simulink model "SinglePhase_NLCurrent_compensation"  (R2017b)
settings: Solver=ode4  StartTime=0.0  StopTime=simend  FixedStep=ts  RelTol=1e-3
values from neighbouring files (symbols this model uses):
  B = BT(:,1:size(B1,2))    [SinglePhase_NLCurrent_compensation_parameter.m]
  gamma = zeros(Hp*n,Hp*d)    [mpc_matrixSetup.m]
  hp = num    (= 1000)    [SinglePhase_NLCurrent_compensation_parameter.m]
  hu = hp    (= 1000)    [SinglePhase_NLCurrent_compensation_parameter.m]
  mtd = 3    [SinglePhase_NLCurrent_compensation_parameter.m]
  num = 1000    [SinglePhase_NLCurrent_compensation_parameter.m]
  psi = zeros(Hp*n,n)    [mpc_matrixSetup.m]
  Q = QPv    [SinglePhase_NLCurrent_compensation_parameter.m]
  R = 1*10^(+5-0)*eye(hu*size(B,2))    [SinglePhase_NLCurrent_compensation_parameter.m]
  ref = ref(:)    [SinglePhase_NLCurrent_compensation_parameter.m]
  Rline = 1    [SinglePhase_NLCurrent_compensation_parameter.m]
  SQ = Pv    [SinglePhase_NLCurrent_compensation_parameter.m]
  SR = chol(R)    [SinglePhase_NLCurrent_compensation_parameter.m]
  theta = zeros(Hp*n,Hu*m)    [mpc_matrixSetup.m]
  ts = 1/f/num    (= 2e-05)    [SinglePhase_NLCurrent_compensation_parameter.m]
  ups = zeros(Hp*n,m)    [mpc_matrixSetup.m]
undefined symbols (not defined in the file or in its folder): A
libraries: fl_lib x37, nesl_utility x21, simulink x4, powerlib_meascontrol x1
settings Model: PauseTimes=0.02  Creator=Weihe  LastModifiedBy=Weihe

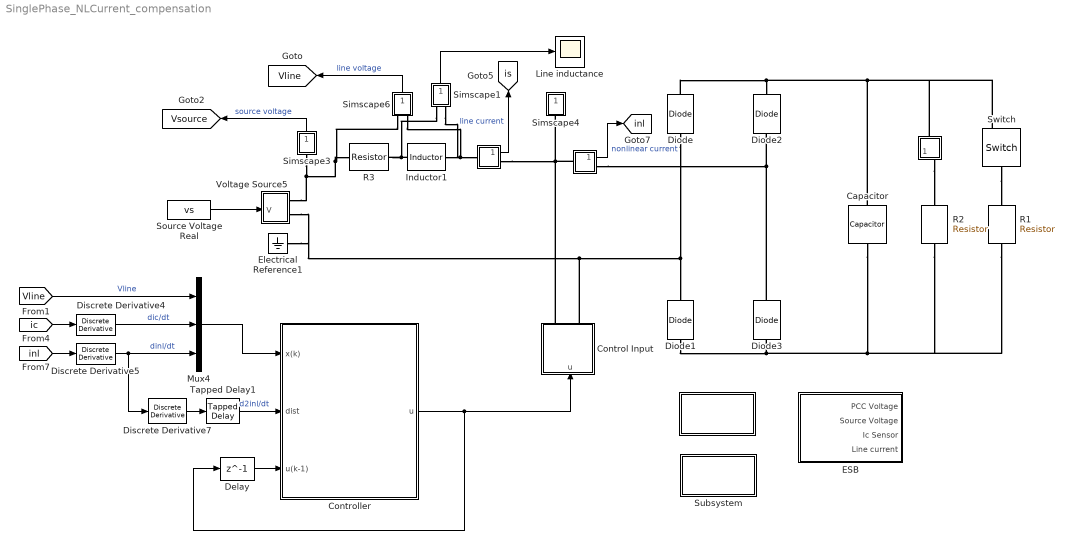
== system SinglePhase_NLCurrent_compensation ==
  " " : Subsystem
      mask Display: disp('A')
  "     " : Subsystem
      mask Display: disp('A')
  "      " : Subsystem
      mask Display: disp('A')
  "           " : Subsystem
      mask Display: disp('THD Calculation')
  Capacitor : fl_lib/Electrical/Electrical Elements/Capacitor  c=5e-3 F  r=1e-6 Ohm  g=0 1/Ohm  i_specify=off  i_priority=None  i=0 A  i_nominal_specify=off  i_nominal_unit=A  i_nominal_value=1  v_specify=off  v_priority=None  v=0 V  v_nominal_specify=off  v_nominal_unit=V  v_nominal_value=1  vc_specify=off  vc_priority=High  vc=0 V  vc_nominal_specify=off  vc_nominal_unit=V  vc_nominal_value=1
  Control Input : Subsystem
  Controller : Subsystem
  Delay : Delay  DelayLength=1
  Diode{,1..3} (4 alike) : fl_lib/Electrical/Electrical Elements/Diode  Vf=0.6 V  Ron=0.3 Ohm  Goff=1e-8 1/Ohm  i_specify=off  i_priority=None  i=0 A  i_nominal_specify=off  i_nominal_unit=A  i_nominal_value=1  v_specify=off  v_priority=None  v=0 V  v_nominal_specify=off  v_nominal_unit=V  v_nominal_value=1
  Discrete Derivative4 : simulink/Discrete/Discrete Derivative  gainval=1e-0  ICPrevScaledInput=0.0  OutMin=[]  OutMax=[]  OutDataType=fixdt(1, 16)  OutScaling=2^-10  DoSatur=off
  Discrete Derivative5 : simulink/Discrete/Discrete Derivative  gainval=1e-0  ICPrevScaledInput=0.0  OutMin=[]  OutMax=[]  OutDataType=fixdt(1, 16)  OutScaling=2^-10  DoSatur=off
  Discrete Derivative7 : simulink/Discrete/Discrete Derivative  gainval=1.0  ICPrevScaledInput=0.0  OutMin=[]  OutMax=[]  OutDataType=fixdt(1, 16)  OutScaling=2^-10  DoSatur=off
  ESB : Subsystem
  Electrical Reference1 : fl_lib/Electrical/Electrical Elements/Electrical Reference
  Inductor1 : fl_lib/Electrical/Electrical Elements/Inductor  l=Lline H  r=0 Ohm  g=1e-9 1/Ohm  i_specify=off  i_priority=None  i=0 A  i_nominal_specify=off  i_nominal_unit=A  i_nominal_value=1  v_specify=off  v_priority=None  v=0 V  v_nominal_specify=off  v_nominal_unit=V  v_nominal_value=1  i_L_specify=off  i_L_priority=High  i_L=0 A  i_L_nominal_specify=off  i_L_nominal_unit=A  i_L_nominal_value=1
  Line inductance : Scope
  Mux4 : Mux  Inputs=3
  R1 : fl_lib/Electrical/Electrical Elements/Resistor  R=10 Ohm  i_specify=off  i_priority=High  i=0 A  i_nominal_specify=off  i_nominal_unit=A  i_nominal_value=1  v_specify=off  v_priority=High  v=0 V  v_nominal_specify=off  v_nominal_unit=V  v_nominal_value=1
  R2 : fl_lib/Electrical/Electrical Elements/Resistor  R=10 Ohm  i_specify=off  i_priority=High  i=0 A  i_nominal_specify=off  i_nominal_unit=A  i_nominal_value=1  v_specify=off  v_priority=High  v=0 V  v_nominal_specify=off  v_nominal_unit=V  v_nominal_value=1
  R3 : fl_lib/Electrical/Electrical Elements/Resistor  R=Rline Ohm  i_specify=off  i_priority=High  i=0 A  i_nominal_specify=off  i_nominal_unit=A  i_nominal_value=1  v_specify=off  v_priority=High  v=0 V  v_nominal_specify=off  v_nominal_unit=V  v_nominal_value=1
  Simscape1 : Subsystem
      mask Display: disp('V')
  Simscape3 : Subsystem
      mask Display: disp('V')
  Simscape4 : Subsystem
      mask Display: disp('V')
  Simscape6 : Subsystem
      mask Display: disp('V')
  Source Voltage Real : FromWorkspace  VariableName=vs  SampleTime=ts  Interpolate=off  OutputAfterFinalValue=Holding final value
  Subsystem : Subsystem
      mask Display: disp('Scopes')
  Switch : fl_lib/Electrical/Electrical Elements/Switch  R_closed=0.01 Ohm  G_open=1e-8 1/Ohm  Threshold=0  i_specify=off  i_priority=None  i=0 A  i_nominal_specify=off  i_nominal_unit=A  i_nominal_value=1  v_specify=off  v_priority=None  v=0 V  v_nominal_specify=off  v_nominal_unit=V  v_nominal_value=1
      settings: SourceProductName=Simscape
  Tapped Delay1 : simulink/Discrete/Tapped Delay  vinit=0.0  samptime=ts  NumDelays=num  DelayOrder=Oldest  includeCurrent=off
  Voltage Source5 : Subsystem
  tag scope: Vline=global, Vsource=global, inl=global, is=global
  wires:
  Source Voltage Real/1 -> Voltage Source5/1(V)
  " "/1(Out1) -> [is]  "line current"
  Discrete Derivative4/1 -> Mux4/2  "dic/dt"
  Discrete Derivative5/1 -> Discrete Derivative7/1, Mux4/3  "dinl/dt"
  "      "/1(Out1) -> [inl]  "nonlinear current"
  Controller/1(u) -> Control Input/1(u), Delay/1
  Mux4/1 -> Controller/1(x(k))
  Tapped Delay1/1 -> Controller/2(dist)  "d2inl/dt"
  Delay/1 -> Controller/3(u(k-1))
  Discrete Derivative7/1 -> Tapped Delay1/1
  Simscape6/1(Out) -> [Vline]  "line voltage"
  [Vline] -> Mux4/1  "Vline"
  [ic] -> Discrete Derivative4/1
  [inl] -> Discrete Derivative5/1
  Simscape3/1(Out) -> [Vsource]  "source voltage"
  Simscape1/1(Out) -> Line inductance/1
  connections:
  Voltage Source5/RConn1 -- Simscape6/LConn1 -- R3/LConn1 -- Simscape3/LConn1
  Diode/LConn1 -- Diode1/RConn1 -- Control Input/RConn2 -- Electrical Reference1/LConn1 -- Voltage Source5/RConn2
  Diode3/RConn1 -- "      "/RConn1 -- Diode2/LConn1
  Diode/RConn1 -- Switch/RConn2 -- "     "/LConn1 -- Capacitor/LConn1 -- Diode2/RConn1
  Diode1/LConn1 -- R1/RConn1 -- R2/RConn1 -- Capacitor/RConn1 -- Diode3/LConn1
  "     "/RConn1 -- R2/LConn1
  Inductor1/RConn1 -- Simscape1/LConn2 -- Simscape6/LConn2 -- " "/LConn1
  Inductor1/LConn1 -- Simscape1/LConn1 -- R3/RConn1
  "      "/LConn1 -- Control Input/RConn1 -- " "/RConn1 -- Simscape4/LConn1
  Switch/LConn1 -- R1/LConn1

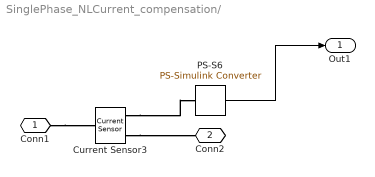
== system SinglePhase_NLCurrent_compensation/  ==
  Current Sensor3 : fl_lib/Electrical/Electrical Sensors/Current Sensor  mask(Current Sensor){}
  PS-S6 : nesl_utility/PS-Simulink Converter  PhysicalDomain=network_engine_domain  SubClassName=ps_output  LeftPortType=input  RightPortType=output  PseudoPeriodic=off  Frequencies=[]  Unit=A  AffineConversion=off
  Conn1 : PMIOPort  Port=1  Side=Left
  Conn2 : PMIOPort  Port=2  Side=Right
  Out1 : Outport
  wires:
  PS-S6/1 -> Out1/1
  connections:
  Current Sensor3/RConn2 -- Conn2/RConn1
  Conn1/RConn1 -- Current Sensor3/LConn1
  Current Sensor3/RConn1 -- PS-S6/LConn1

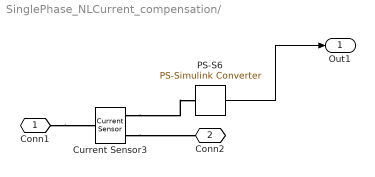
== system SinglePhase_NLCurrent_compensation/      ==
  Current Sensor3 : fl_lib/Electrical/Electrical Sensors/Current Sensor  mask(Current Sensor){}
  PS-S6 : nesl_utility/PS-Simulink Converter  PhysicalDomain=network_engine_domain  SubClassName=ps_output  LeftPortType=input  RightPortType=output  PseudoPeriodic=off  Frequencies=[]  Unit=A  AffineConversion=off
  Conn1 : PMIOPort  Port=1  Side=Left
  Conn2 : PMIOPort  Port=2  Side=Right
  Out1 : Outport
  wires:
  PS-S6/1 -> Out1/1
  connections:
  Current Sensor3/RConn2 -- Conn2/RConn1
  Conn1/RConn1 -- Current Sensor3/LConn1
  Current Sensor3/RConn1 -- PS-S6/LConn1

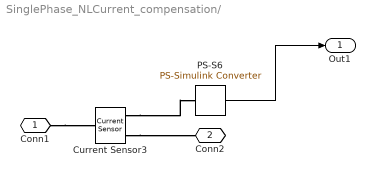
== system SinglePhase_NLCurrent_compensation/       ==
  Current Sensor3 : fl_lib/Electrical/Electrical Sensors/Current Sensor  mask(Current Sensor){}
  PS-S6 : nesl_utility/PS-Simulink Converter  PhysicalDomain=network_engine_domain  SubClassName=ps_output  LeftPortType=input  RightPortType=output  PseudoPeriodic=off  Frequencies=[]  Unit=A  AffineConversion=off
  Conn1 : PMIOPort  Port=1  Side=Left
  Conn2 : PMIOPort  Port=2  Side=Right
  Out1 : Outport
  wires:
  PS-S6/1 -> Out1/1
  connections:
  Current Sensor3/RConn2 -- Conn2/RConn1
  Conn1/RConn1 -- Current Sensor3/LConn1
  Current Sensor3/RConn1 -- PS-S6/LConn1

== system SinglePhase_NLCurrent_compensation/            ==
  Display : Display
  THD : powerlib_meascontrol/Measurements/THD  Freq=f  Ts=ts
  THD Vline : Scope
  wires:
  THD/1 -> Display/1, THD Vline/1
  [is] -> THD/1

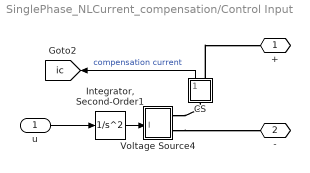
== system SinglePhase_NLCurrent_compensation/Control Input ==
  u : Inport
  CS : Subsystem
      mask Display: disp('A')
  "Integrator, Second-Order1" : SecondOrderIntegrator  ShowOutput=x
  Voltage Source4 : Subsystem
  + : PMIOPort  Port=1  Side=Right
  - : PMIOPort  Port=2  Side=Right
  tag scope: ic=global
  wires:
  "Integrator, Second-Order1"/1 -> Voltage Source4/1(I)
  u/1 -> "Integrator, Second-Order1"/1
  CS/1(Out1) -> [ic]  "compensation current"
  connections:
  Voltage Source4/RConn1 -- CS/LConn1
  CS/RConn1 -- +/RConn1
  Voltage Source4/RConn2 -- -/RConn1

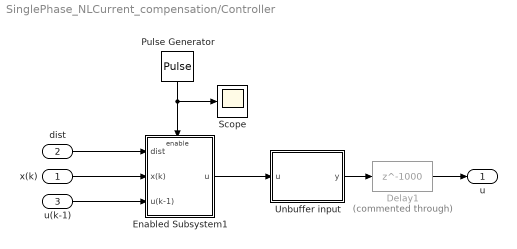
== system SinglePhase_NLCurrent_compensation/Controller ==
  x(k) : Inport
  dist : Inport  Port=2
  u(k-1) : Inport  Port=3
  Delay1 : Delay  Commented=through  DelayLength=1000
  Enabled Subsystem1 : Subsystem  TreatAsAtomicUnit=on
  Pulse Generator : DiscretePulseGenerator  Period=num  SampleTime=ts
  Scope : Scope
  Unbuffer input : MATLAB Function  TreatAsAtomicUnit=on  SystemSampleTime=ts
  u : Outport
  wires:
  Pulse Generator/1 -> Enabled Subsystem1/Enable, Scope/1
  dist/1 -> Enabled Subsystem1/1(dist)
  Delay1/1 -> u/1
  x(k)/1 -> Enabled Subsystem1/2(x(k))
  u(k-1)/1 -> Enabled Subsystem1/3(u(k-1))
  Enabled Subsystem1/1(u) -> Unbuffer input/1(u)
  Unbuffer input/1(y) -> Delay1/1

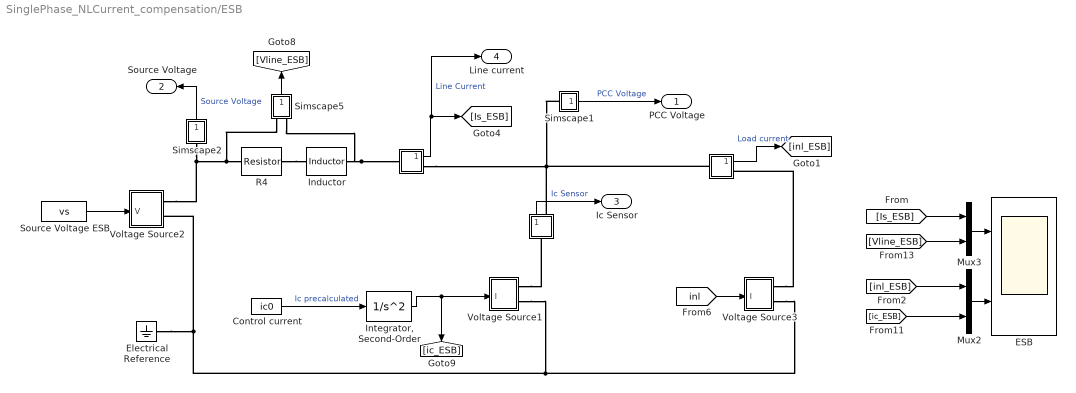
== system SinglePhase_NLCurrent_compensation/ESB ==
  "  " : Subsystem
      mask Display: disp('A')
  "   " : Subsystem
      mask Display: disp('A')
  "    " : Subsystem
      mask Display: disp('A')
  Control current : FromWorkspace  VariableName=ic0  SampleTime=ts  Interpolate=off  OutputAfterFinalValue=Holding final value
  ESB : Scope  NumInputPorts=2
  Electrical Reference : fl_lib/Electrical/Electrical Elements/Electrical Reference
  Inductor : fl_lib/Electrical/Electrical Elements/Inductor  l=Lline H  r=0 Ohm  g=1e-9 1/Ohm  i_specify=off  i_priority=None  i=0 A  i_nominal_specify=off  i_nominal_unit=A  i_nominal_value=1  v_specify=off  v_priority=None  v=0 V  v_nominal_specify=off  v_nominal_unit=V  v_nominal_value=1  i_L_specify=off  i_L_priority=High  i_L=0 A  i_L_nominal_specify=off  i_L_nominal_unit=A  i_L_nominal_value=1
  "Integrator, Second-Order" : SecondOrderIntegrator  ShowOutput=x
  Mux2 : Mux  Inputs=2
  Mux3 : Mux  Inputs=2
  R4 : fl_lib/Electrical/Electrical Elements/Resistor  R=Rline Ohm  i_specify=off  i_priority=High  i=0 A  i_nominal_specify=off  i_nominal_unit=A  i_nominal_value=1  v_specify=off  v_priority=High  v=0 V  v_nominal_specify=off  v_nominal_unit=V  v_nominal_value=1
  Simscape1 : Subsystem
      mask Display: disp('V')
  Simscape2 : Subsystem
      mask Display: disp('V')
  Simscape5 : Subsystem
      mask Display: disp('V')
  Source Voltage ESB : FromWorkspace  VariableName=vs  SampleTime=ts  Interpolate=off  OutputAfterFinalValue=Holding final value
  Voltage Source1 : Subsystem
  Voltage Source2 : Subsystem
  Voltage Source3 : Subsystem
  PCC Voltage : Outport
  Source Voltage : Outport  Port=2
  Ic Sensor : Outport  Port=3
  Line current : Outport  Port=4
  wires:
  "  "/1(Out1) -> [inl_ESB]  "Load current"
  "   "/1(Out1) -> Line current/1, [Is_ESB]  "Line Current"
  Source Voltage ESB/1 -> Voltage Source2/1(V)
  Simscape5/1(Out) -> [Vline_ESB]
  [ic_ESB] -> Mux2/2
  [inl_ESB] -> Mux2/1
  [inl] -> Voltage Source3/1(I)
  "Integrator, Second-Order"/1 -> Voltage Source1/1(I), [ic_ESB]
  Mux3/1 -> ESB/1
  [Is_ESB] -> Mux3/1
  [Vline_ESB] -> Mux3/2
  Control current/1 -> "Integrator, Second-Order"/1  "Ic precalculated"
  Mux2/1 -> ESB/2
  "    "/1(Out1) -> Ic Sensor/1  "Ic Sensor"
  Simscape1/1(Out) -> PCC Voltage/1  "PCC Voltage"
  Simscape2/1(Out) -> Source Voltage/1  "Source Voltage"
  connections:
  Voltage Source1/RConn2 -- Voltage Source3/RConn2 -- Electrical Reference/LConn1 -- Voltage Source2/RConn2
  Voltage Source2/RConn1 -- Simscape5/LConn1 -- R4/LConn1 -- Simscape2/LConn1
  Voltage Source1/RConn1 -- "    "/LConn1
  "    "/RConn1 -- "  "/LConn1 -- "   "/RConn1 -- Simscape1/LConn1
  Voltage Source3/RConn1 -- "  "/RConn1
  Inductor/RConn1 -- Simscape5/LConn2 -- "   "/LConn1
  R4/RConn1 -- Inductor/LConn1

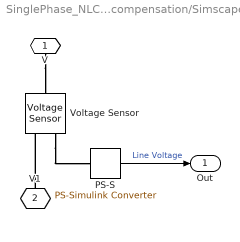
== system SinglePhase_NLCurrent_compensation/Simscape1 ==
  PS-S : nesl_utility/PS-Simulink Converter  PhysicalDomain=network_engine_domain  SubClassName=ps_output  LeftPortType=input  RightPortType=output  PseudoPeriodic=off  Frequencies=[]  Unit=V  AffineConversion=off
  Voltage Sensor : fl_lib/Electrical/Electrical Sensors/Voltage Sensor
  V : PMIOPort  Port=1  Side=Left
  V1 : PMIOPort  Port=2  Side=Left
  Out : Outport
  wires:
  PS-S/1 -> Out/1  "Line Voltage"
  connections:
  V/RConn1 -- Voltage Sensor/LConn1
  V1/RConn1 -- Voltage Sensor/RConn2
  Voltage Sensor/RConn1 -- PS-S/LConn1

== system SinglePhase_NLCurrent_compensation/Simscape3 ==
  Electrical Reference1 : fl_lib/Electrical/Electrical Elements/Electrical Reference
  PS-S : nesl_utility/PS-Simulink Converter  PhysicalDomain=network_engine_domain  SubClassName=ps_output  LeftPortType=input  RightPortType=output  PseudoPeriodic=off  Frequencies=[]  Unit=V  AffineConversion=off
  Voltage Sensor : fl_lib/Electrical/Electrical Sensors/Voltage Sensor
  V : PMIOPort  Port=1  Side=Left
  Out : Outport
  wires:
  PS-S/1 -> Out/1  "voltage"
  connections:
  V/RConn1 -- Voltage Sensor/LConn1
  Electrical Reference1/LConn1 -- Voltage Sensor/RConn2
  Voltage Sensor/RConn1 -- PS-S/LConn1

== system SinglePhase_NLCurrent_compensation/Simscape4 ==
  Electrical Reference1 : fl_lib/Electrical/Electrical Elements/Electrical Reference
  PS-S : nesl_utility/PS-Simulink Converter  PhysicalDomain=network_engine_domain  SubClassName=ps_output  LeftPortType=input  RightPortType=output  PseudoPeriodic=off  Frequencies=[]  Unit=V  AffineConversion=off
  Voltage Sensor : fl_lib/Electrical/Electrical Sensors/Voltage Sensor
  V : PMIOPort  Port=1  Side=Left
  Out : Outport
  wires:
  PS-S/1 -> Out/1  "voltage"
  connections:
  PS-S/LConn1 -- Voltage Sensor/RConn1
  V/RConn1 -- Voltage Sensor/LConn1
  Electrical Reference1/LConn1 -- Voltage Sensor/RConn2

== system SinglePhase_NLCurrent_compensation/Simscape6 ==
  PS-S : nesl_utility/PS-Simulink Converter  PhysicalDomain=network_engine_domain  SubClassName=ps_output  LeftPortType=input  RightPortType=output  PseudoPeriodic=off  Frequencies=[]  Unit=V  AffineConversion=off
  Voltage Sensor : fl_lib/Electrical/Electrical Sensors/Voltage Sensor
  V : PMIOPort  Port=1  Side=Left
  V1 : PMIOPort  Port=2  Side=Left
  Out : Outport
  wires:
  PS-S/1 -> Out/1  "Line Voltage"
  connections:
  V/RConn1 -- Voltage Sensor/LConn1
  V1/RConn1 -- Voltage Sensor/RConn2
  Voltage Sensor/RConn1 -- PS-S/LConn1

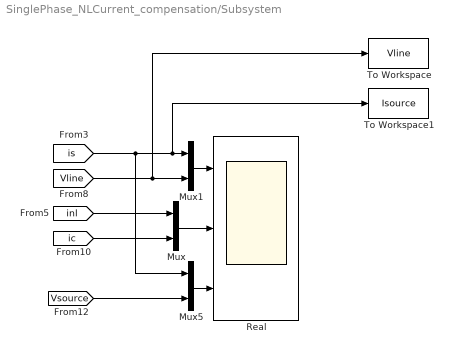
== system SinglePhase_NLCurrent_compensation/Subsystem ==
  Mux : Mux  Inputs=2
  Mux1 : Mux  Inputs=2
  Mux5 : Mux  Inputs=2
  Real : Scope  NumInputPorts=3
  To Workspace : ToWorkspace  VariableName=Vline  SaveFormat=Structure  SampleTime=-1
  To Workspace1 : ToWorkspace  VariableName=Isource  SaveFormat=Structure  SampleTime=-1
  wires:
  [inl] -> Mux/1
  [ic] -> Mux/2
  [Vline] -> To Workspace/1, Mux1/2
  [Vsource] -> Mux5/2
  Mux5/1 -> Real/3
  [is] -> Mux5/1, To Workspace1/1, Mux1/1
  Mux1/1 -> Real/1
  Mux/1 -> Real/2

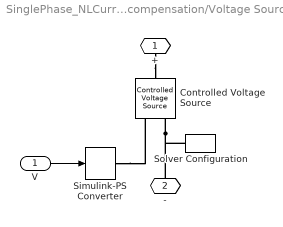
== system SinglePhase_NLCurrent_compensation/Voltage Source5 ==
  V : Inport
  Controlled Voltage Source : fl_lib/Electrical/Electrical Sources/Controlled Voltage Source
  Simulink-PS Converter : nesl_utility/Simulink-PS Converter  PhysicalDomain=network_engine_domain  SubClassName=ps_input  LeftPortType=input  RightPortType=output  PseudoPeriodic=off  Frequencies=[]  NoiseDistribution=none  NoiseParameters=[]  Unit=1  AffineConversion=off  FilteringAndDerivatives=zero  SimscapeFilterOrder=1  InputFilterTimeConstant=.001  UdotUserProvided=0
  Solver Configuration : nesl_utility/Solver Configuration  PhysicalDomain=network_engine_domain  SubClassName=solver  LeftPortType=input  RightPortType=generic  Accelerate=off  Tones=[]  Harmonics=[]  SimulateNoise=off  Profile=off  UseLocalSampling=off  EnableSwitchedLinearOptims=on  FrequencyDomain=off  UseCCode=off  RelTol=0.001  AbsTol=1e-06  MinStep=1e-09  ToWorkspace=off  RevertToSquareIcSolve=off  NumHomotopyIterations=100  PhasorMode=off  PhasorModeNumHarmonics=1  DoDC=off  ResidualTolerance=1e-9  UseLocalSolver=on  LocalSolverChoice=NE_BACKWARD_EULER_ADVANCER  LocalSolverSampleTime=ts  DoFixedCost=on  MaxNonlinIter=3  MaxModeIter=2  LinearAlgebra=Sparse  DelaysMemoryBudget=1024  AutomaticFiltering=off  FilteringTimeConstant=0.001
  + : PMIOPort  Port=1  Side=Right
  - : PMIOPort  Port=2  Side=Right
  wires:
  V/1 -> Simulink-PS Converter/1
  connections:
  Simulink-PS Converter/RConn1 -- Controlled Voltage Source/RConn1
  Controlled Voltage Source/RConn2 -- -/RConn1 -- Solver Configuration/RConn1
  +/RConn1 -- Controlled Voltage Source/LConn1

== system SinglePhase_NLCurrent_compensation/Control Input/CS ==
  Current Sensor3 : fl_lib/Electrical/Electrical Sensors/Current Sensor  mask(Current Sensor){}
  PS-S6 : nesl_utility/PS-Simulink Converter  PhysicalDomain=network_engine_domain  SubClassName=ps_output  LeftPortType=input  RightPortType=output  PseudoPeriodic=off  Frequencies=[]  Unit=A  AffineConversion=off
  Conn1 : PMIOPort  Port=1  Side=Left
  Conn2 : PMIOPort  Port=2  Side=Right
  Out1 : Outport
  wires:
  PS-S6/1 -> Out1/1
  connections:
  Current Sensor3/RConn2 -- Conn2/RConn1
  Conn1/RConn1 -- Current Sensor3/LConn1
  Current Sensor3/RConn1 -- PS-S6/LConn1

== system SinglePhase_NLCurrent_compensation/Control Input/Voltage Source4 ==
  I : Inport
  Controlled Current Source : fl_lib/Electrical/Electrical Sources/Controlled Current Source
  Simulink-PS Converter : nesl_utility/Simulink-PS Converter  PhysicalDomain=network_engine_domain  SubClassName=ps_input  LeftPortType=input  RightPortType=output  PseudoPeriodic=off  Frequencies=[]  NoiseDistribution=none  NoiseParameters=[]  Unit=1  AffineConversion=off  FilteringAndDerivatives=zero  SimscapeFilterOrder=1  InputFilterTimeConstant=.001  UdotUserProvided=0
  + : PMIOPort  Port=1  Side=Right
  - : PMIOPort  Port=2  Side=Right
  wires:
  I/1 -> Simulink-PS Converter/1
  connections:
  Controlled Current Source/RConn1 -- Simulink-PS Converter/RConn1
  -/RConn1 -- Controlled Current Source/RConn2
  Controlled Current Source/LConn1 -- +/RConn1

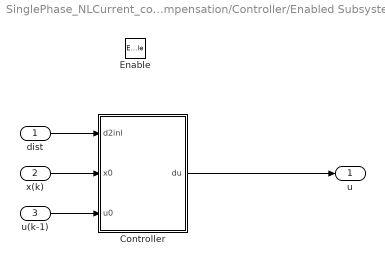
== system SinglePhase_NLCurrent_compensation/Controller/Enabled Subsystem1 ==
  dist : Inport
  x(k) : Inport  Port=2
  u(k-1) : Inport  Port=3
  Enable : EnablePort  PropagateVarSize=During execution
  Controller : MATLAB Function  TreatAsAtomicUnit=on  SystemSampleTime=ts
  u : Outport
  wires:
  dist/1 -> Controller/1(d2inl)
  x(k)/1 -> Controller/2(x0)
  u(k-1)/1 -> Controller/3(u0)
  Controller/1(du) -> u/1

== system SinglePhase_NLCurrent_compensation/ESB/   ==
  Current Sensor3 : fl_lib/Electrical/Electrical Sensors/Current Sensor  mask(Current Sensor){}
  PS-S6 : nesl_utility/PS-Simulink Converter  PhysicalDomain=network_engine_domain  SubClassName=ps_output  LeftPortType=input  RightPortType=output  PseudoPeriodic=off  Frequencies=[]  Unit=A  AffineConversion=off
  Conn1 : PMIOPort  Port=1  Side=Left
  Conn2 : PMIOPort  Port=2  Side=Right
  Out1 : Outport
  wires:
  PS-S6/1 -> Out1/1
  connections:
  Current Sensor3/RConn2 -- Conn2/RConn1
  Conn1/RConn1 -- Current Sensor3/LConn1
  Current Sensor3/RConn1 -- PS-S6/LConn1

== system SinglePhase_NLCurrent_compensation/ESB/    ==
  Current Sensor3 : fl_lib/Electrical/Electrical Sensors/Current Sensor  mask(Current Sensor){}
  PS-S6 : nesl_utility/PS-Simulink Converter  PhysicalDomain=network_engine_domain  SubClassName=ps_output  LeftPortType=input  RightPortType=output  PseudoPeriodic=off  Frequencies=[]  Unit=A  AffineConversion=off
  Conn1 : PMIOPort  Port=1  Side=Left
  Conn2 : PMIOPort  Port=2  Side=Right
  Out1 : Outport
  wires:
  PS-S6/1 -> Out1/1
  connections:
  Current Sensor3/RConn2 -- Conn2/RConn1
  Conn1/RConn1 -- Current Sensor3/LConn1
  Current Sensor3/RConn1 -- PS-S6/LConn1

== system SinglePhase_NLCurrent_compensation/ESB/     ==
  Current Sensor3 : fl_lib/Electrical/Electrical Sensors/Current Sensor  mask(Current Sensor){}
  PS-S6 : nesl_utility/PS-Simulink Converter  PhysicalDomain=network_engine_domain  SubClassName=ps_output  LeftPortType=input  RightPortType=output  PseudoPeriodic=off  Frequencies=[]  Unit=A  AffineConversion=off
  Conn1 : PMIOPort  Port=1  Side=Left
  Conn2 : PMIOPort  Port=2  Side=Right
  Out1 : Outport
  wires:
  PS-S6/1 -> Out1/1
  connections:
  Current Sensor3/RConn2 -- Conn2/RConn1
  Conn1/RConn1 -- Current Sensor3/LConn1
  Current Sensor3/RConn1 -- PS-S6/LConn1

== system SinglePhase_NLCurrent_compensation/ESB/Simscape1 ==
  Electrical Reference1 : fl_lib/Electrical/Electrical Elements/Electrical Reference
  PS-S : nesl_utility/PS-Simulink Converter  PhysicalDomain=network_engine_domain  SubClassName=ps_output  LeftPortType=input  RightPortType=output  PseudoPeriodic=off  Frequencies=[]  Unit=V  AffineConversion=off
  Voltage Sensor : fl_lib/Electrical/Electrical Sensors/Voltage Sensor
  V : PMIOPort  Port=1  Side=Left
  Out : Outport
  wires:
  PS-S/1 -> Out/1  "voltage"
  connections:
  PS-S/LConn1 -- Voltage Sensor/RConn1
  V/RConn1 -- Voltage Sensor/LConn1
  Electrical Reference1/LConn1 -- Voltage Sensor/RConn2

== system SinglePhase_NLCurrent_compensation/ESB/Simscape2 ==
  Electrical Reference1 : fl_lib/Electrical/Electrical Elements/Electrical Reference
  PS-S : nesl_utility/PS-Simulink Converter  PhysicalDomain=network_engine_domain  SubClassName=ps_output  LeftPortType=input  RightPortType=output  PseudoPeriodic=off  Frequencies=[]  Unit=V  AffineConversion=off
  Voltage Sensor : fl_lib/Electrical/Electrical Sensors/Voltage Sensor
  V : PMIOPort  Port=1  Side=Left
  Out : Outport
  wires:
  PS-S/1 -> Out/1  "voltage"
  connections:
  V/RConn1 -- Voltage Sensor/LConn1
  Electrical Reference1/LConn1 -- Voltage Sensor/RConn2
  Voltage Sensor/RConn1 -- PS-S/LConn1

== system SinglePhase_NLCurrent_compensation/ESB/Simscape5 ==
  PS-S : nesl_utility/PS-Simulink Converter  PhysicalDomain=network_engine_domain  SubClassName=ps_output  LeftPortType=input  RightPortType=output  PseudoPeriodic=off  Frequencies=[]  Unit=V  AffineConversion=off
  Voltage Sensor : fl_lib/Electrical/Electrical Sensors/Voltage Sensor
  V : PMIOPort  Port=1  Side=Left
  V1 : PMIOPort  Port=2  Side=Left
  Out : Outport
  wires:
  PS-S/1 -> Out/1  "Line Voltage"
  connections:
  V/RConn1 -- Voltage Sensor/LConn1
  V1/RConn1 -- Voltage Sensor/RConn2
  Voltage Sensor/RConn1 -- PS-S/LConn1

== system SinglePhase_NLCurrent_compensation/ESB/Voltage Source1 ==
  I : Inport
  Controlled Current Source : fl_lib/Electrical/Electrical Sources/Controlled Current Source
  Simulink-PS Converter : nesl_utility/Simulink-PS Converter  PhysicalDomain=network_engine_domain  SubClassName=ps_input  LeftPortType=input  RightPortType=output  PseudoPeriodic=off  Frequencies=[]  NoiseDistribution=none  NoiseParameters=[]  Unit=1  AffineConversion=off  FilteringAndDerivatives=zero  SimscapeFilterOrder=1  InputFilterTimeConstant=.001  UdotUserProvided=0
  + : PMIOPort  Port=1  Side=Right
  - : PMIOPort  Port=2  Side=Right
  wires:
  I/1 -> Simulink-PS Converter/1
  connections:
  Controlled Current Source/RConn1 -- Simulink-PS Converter/RConn1
  -/RConn1 -- Controlled Current Source/RConn2
  Controlled Current Source/LConn1 -- +/RConn1

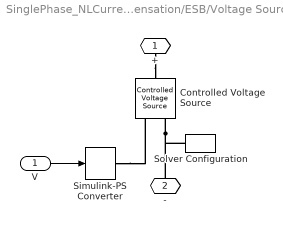
== system SinglePhase_NLCurrent_compensation/ESB/Voltage Source2 ==
  V : Inport
  Controlled Voltage Source : fl_lib/Electrical/Electrical Sources/Controlled Voltage Source
  Simulink-PS Converter : nesl_utility/Simulink-PS Converter  PhysicalDomain=network_engine_domain  SubClassName=ps_input  LeftPortType=input  RightPortType=output  PseudoPeriodic=off  Frequencies=[]  NoiseDistribution=none  NoiseParameters=[]  Unit=1  AffineConversion=off  FilteringAndDerivatives=zero  SimscapeFilterOrder=1  InputFilterTimeConstant=.001  UdotUserProvided=0
  Solver Configuration : nesl_utility/Solver Configuration  PhysicalDomain=network_engine_domain  SubClassName=solver  LeftPortType=input  RightPortType=generic  Accelerate=off  Tones=[]  Harmonics=[]  SimulateNoise=off  Profile=off  UseLocalSampling=off  EnableSwitchedLinearOptims=on  FrequencyDomain=off  UseCCode=off  RelTol=0.001  AbsTol=1e-06  MinStep=1e-09  ToWorkspace=off  RevertToSquareIcSolve=off  NumHomotopyIterations=100  PhasorMode=off  PhasorModeNumHarmonics=1  DoDC=off  ResidualTolerance=1e-9  UseLocalSolver=on  LocalSolverChoice=NE_BACKWARD_EULER_ADVANCER  LocalSolverSampleTime=ts  DoFixedCost=on  MaxNonlinIter=3  MaxModeIter=2  LinearAlgebra=Sparse  DelaysMemoryBudget=1024  AutomaticFiltering=off  FilteringTimeConstant=0.001
  + : PMIOPort  Port=1  Side=Right
  - : PMIOPort  Port=2  Side=Right
  wires:
  V/1 -> Simulink-PS Converter/1
  connections:
  Simulink-PS Converter/RConn1 -- Controlled Voltage Source/RConn1
  Controlled Voltage Source/RConn2 -- -/RConn1 -- Solver Configuration/RConn1
  +/RConn1 -- Controlled Voltage Source/LConn1

== system SinglePhase_NLCurrent_compensation/ESB/Voltage Source3 ==
  I : Inport
  Controlled Current Source : fl_lib/Electrical/Electrical Sources/Controlled Current Source
  Simulink-PS Converter : nesl_utility/Simulink-PS Converter  PhysicalDomain=network_engine_domain  SubClassName=ps_input  LeftPortType=input  RightPortType=output  PseudoPeriodic=off  Frequencies=[]  NoiseDistribution=none  NoiseParameters=[]  Unit=1  AffineConversion=off  FilteringAndDerivatives=zero  SimscapeFilterOrder=1  InputFilterTimeConstant=.001  UdotUserProvided=0
  - : PMIOPort  Port=1  Side=Right
  " +" : PMIOPort  Port=2  Side=Right
  wires:
  I/1 -> Simulink-PS Converter/1
  connections:
  Controlled Current Source/RConn1 -- Simulink-PS Converter/RConn1
  -/RConn1 -- Controlled Current Source/RConn2
  " +"/RConn1 -- Controlled Current Source/LConn1

== matlab function SinglePhase_NLCurrent_compensation/Controller/Unbuffer input ==
  data: u input size=num; y output; hp parameter
function y = unbuffer(u,hp)
%#codegen
persistent count;
if isempty(count)
   count=1; 
end

if count==hp+1
   count=1; 
end

y = u(count);
count=count+1;

== matlab function SinglePhase_NLCurrent_compensation/Controller/Enabled Subsystem1/Controller ==
  data: d2inl input; du output size=[num]; A parameter; B parameter; ref parameter; hp parameter; hu parameter; R parameter; Q parameter; SR parameter; SQ parameter; mtd parameter; x0 input; u0 input; psi parameter; ups parameter; theta parameter; gamma parameter
function du = lsssmpc(d2inl,A,B,ref,hp,hu,R,Q,SR,SQ,mtd,x0,u0,psi,ups,theta,gamma)
%#codegen

n = size(A,1);             % System order
m = size(B,2);             % Number of inputs
E=ref((n+1):n+hp*n)-psi*(A*x0+B*u0)-ups*u0-gamma*d2inl; % Tracking error

switch mtd      % Solution method

    case 2      % Cholesky for Q&R
        SQ=chol(Q);                   % Cholesky deocmposition of Matrix Q
        SR=chol(R);                   % Cholesky deocmposition of Matrix R
        DU=[(SQ*theta);SR]\[(SQ*E);zeros(size(SR,1),size(E,2))];% Optimal input                                 
    case 3      % Custom decomposition
        DU=[(SQ*theta);SR]\[(SQ*E);zeros(size(SR,1),size(E,2))];% Optimal input
     otherwise   % Inverse
        H = theta'*Q*theta+R;         % Matrix H
        G = 2*theta'*Q*E;             % Matrix G
        DU = 0.5 * inv(H) * G;        % Optimal input     
end

du = u0+cumsum([DU ;zeros(hp-hu,m)]);                                  % absolute values of input
